simulink model "fdctools"  (Simulink 2.09)
settings: Solver=ode45  StartTime=0.0  StopTime=999999  MaxStep=10  RelTol=1e-3  AbsTol=1e-3
settings Model: SaveTime=off  SaveOutput=off  ConsistencyChecking=off  RTWTemplateMakefile=grt_vc.tmf

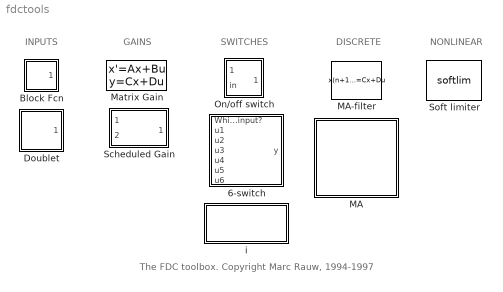
== system fdctools ==
  note: The FDC toolbox. Copyright Marc Rauw, 1994-1997
  note: GAINS
  note: SWITCHES
  note: DISCRETE
  note: NONLINEAR
  note: INPUTS
  6-switch : Subsystem
      mask Display: disp('6 switch:\ny=u(u[1]+1)')
  Block Fcn : Subsystem  mask(Block Fcn){@1=-1, @2=2, @3=1, @4=4}
      mask prompts: @1 "Initial value (=final value):"; @2 "Amplitude of block (+ = step up, - = step down):"; @3 "Start time of block:"; @4 "Stop time of block:"
      mask help: Block Function
      mask init:
      | yinit=@1; yblock=@2; tstart=@3; tstop=@4;
      mask Help: This block implements a block signal.\nDefine the initial (=final) value, the\namplitude of the block (positive\n= upwards, negative=downwards),\nthe start time, and the stop time (must\nbe smaller than the start time).
      mask Display: plot(0,0,100,100,[100,60,60,20,20,0],[50,50,89,89,50,50])
  Doublet : Subsystem  mask(Doublet){@1=1, @2=1, @3=1, @4=1, @5=-1, @6=0}
      mask prompts: @1 "Start time [sec]:"; @2 "Length of time interval 1 [sec]:"; @3 "Length of time interval 2 [sec]:"; @4 "y1:"; @5 "y2:"; @6 "y start (= y final):"
      mask help: Doublet signal.
      mask init:
      | ts1=@1; dt1=@2; dt2=@3; y1=@4; y2=@5; cnst=@6;
      mask Help: This block implements a \ndoublet signal according to: \ny = y1 if \n   tstart <= t < tstart+dt1 \ny = y2 if \n   tstart+dt1 <= t < tstart+dt1+dt2 \ny = y start = y final if \n   t < tstart or t > tstart+dt1+dt2.
      mask Display: plot([0 1 1 2.5 2.5 4 4 5],[0 0 1 1 -1.5 -1.5 0 0])
  MA : Subsystem
      mask Display: disp('MA filter\nwith better\nicon\n\n(double click)')
  MA-filter : DiscreteStateSpace  A=Ama  B=Bma  C=Cma  D=Dma  X0=xinit  SampleTime=Ts  mask(MA-filter){@1=5, @2=0.1, @3=0}
      mask prompts: @1 "Number of samples for averaging:"; @2 "Sample time:"; @3 "Initial value of input signal:"
      mask help: Digital Moving Average filter
      mask init:
      | ns=@1; Ama=[zeros(1,ns);[eye(ns-1) zeros(ns-1,1)]]; Bma=[1; zeros(ns-1,1)]; Cma=1/ns*ones(1,ns); Dma=0; Ts=@2; uinit=@3; xinit=uinit*ones(ns,1);
      mask Help: Digital Moving Average filter. \ny(k) = 1/n * (u(k) + u(k-1) + ... + u(k-ns)) \nwhere ns is the number of samples \nfor averaging (to be specified by \nthe user).
      mask Display: disp('MA')
  Matrix Gain : StateSpace  A=A  B=B  C=C  D=D  X0=0  mask(Matrix Gain){@1=eye(3)}
      mask prompts: @1 "Gain matrix:"
      mask help: Matrix Gain
      mask init:
      | A=[]; B=[]; C=[]; D=@1;
      mask Help: This block implements an matrix gain.\nThe matrix dimensions must be in accordance\nwith the dimension of the inputvector.
      mask Display: disp('y = M*u')
  On/off switch : Subsystem
      mask Type: On/off switch
      mask Description:
      | If input(1) = 1
      |      output = input(2)
      |  else if input(1) = 0
      |      output = 0
      mask Help: On/off switch.
      mask Display: plot(0,0,100,100,[31,31,32,34,34,32,31,31,0],[50,48,47,48,51,53,51,50,50],[100,75,51],[50,50,97]);disp('?')
  Scheduled Gain : Subsystem
      mask Display: plot(0,0,100,100,[0,100,0],[0,50,100]);disp('K(u1)      ')
  Soft limiter : S-Function  FunctionName=softlim  Parameters=max_u, lin_u  mask(Soft limiter){@1=10, @2=10}
      mask prompts: @1 "Limiter range= max. output value= --(min. output value):"; @2 "% of linear range where y=u (linear throughput):"
      mask help: Soft limiter with partly linear throughput
      mask init:
      | max_u=max(@1,1e-16); lin_u=min(0.9999,(max(@2,0)/100))*max_u; uplot=[-5*max_u:0.25*max_u:5*max_u]; for i = 1:length(uplot); yplot(i)=softlim([],[],uplot(i),3,max_u,lin_u); end;
      mask Help: See source-code of SOFTLIM.M or type HELP SOFTLIM at the command-line.
      mask Display: plot(uplot, yplot, max_u*[-5,-1,1,5], max_u*[-1,-1,1,1], 0, -1.3*max_u, 0, 1.2*max_u, max_u*[-5,5], [0,0]);
  i : Subsystem
      settings: OpenFcn=fdchelp('nswitch')
      mask Display: disp('More info\nfor n-switch')

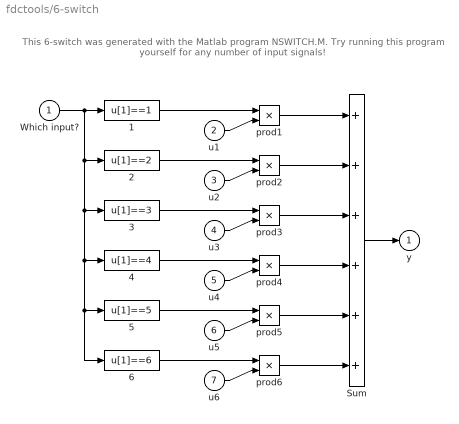
== system fdctools/6-switch ==
  note: This 6-switch was generated with the Matlab program NSWITCH.M.
      | Try running this program yourself for any number of input signals!
  Which input? : Inport  Port=1  PortWidth=-1  SampleTime=-1
  u1 : Inport  Port=2  PortWidth=-1  SampleTime=-1
  u2 : Inport  Port=3  PortWidth=-1  SampleTime=-1
  u3 : Inport  Port=4  PortWidth=-1  SampleTime=-1
  u4 : Inport  Port=5  PortWidth=-1  SampleTime=-1
  u5 : Inport  Port=6  PortWidth=-1  SampleTime=-1
  u6 : Inport  Port=7  PortWidth=-1  SampleTime=-1
  1 : Fcn  Expr=u[1]==1
  2 : Fcn  Expr=u[1]==2
  3 : Fcn  Expr=u[1]==3
  4 : Fcn  Expr=u[1]==4
  5 : Fcn  Expr=u[1]==5
  6 : Fcn  Expr=u[1]==6
  Sum : Sum  Inputs=++++++
  prod{1..6} (6 alike) : Product  Inputs=2
  y : Outport  Port=1  InitialOutput=0
  wires:
  Which input?/1 -> 1/1, 2/1, 3/1, 4/1, 5/1, 6/1
  u1/1 -> prod1/2
  prod1/1 -> Sum/1
  1/1 -> prod1/1
  u2/1 -> prod2/2
  prod2/1 -> Sum/2
  2/1 -> prod2/1
  u3/1 -> prod3/2
  prod3/1 -> Sum/3
  3/1 -> prod3/1
  u4/1 -> prod4/2
  prod4/1 -> Sum/4
  4/1 -> prod4/1
  u5/1 -> prod5/2
  prod5/1 -> Sum/5
  5/1 -> prod5/1
  u6/1 -> prod6/2
  prod6/1 -> Sum/6
  6/1 -> prod6/1
  Sum/1 -> y/1

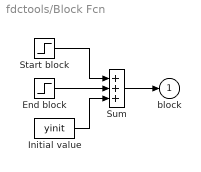
== system fdctools/Block Fcn ==
  End block : Step  Time=tstop  Before=0  After=-yblock
  Initial value : Constant  Value=yinit
  Start block : Step  Time=tstart  Before=0  After=yblock
  Sum : Sum  Inputs=+++
  block : Outport  Port=1  InitialOutput=0
  wires:
  Sum/1 -> block/1
  Initial value/1 -> Sum/3
  Start block/1 -> Sum/1
  End block/1 -> Sum/2

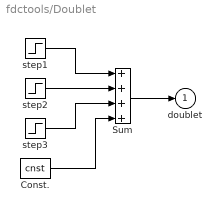
== system fdctools/Doublet ==
  Const. : Constant  Value=cnst
  Sum : Sum  Inputs=++++
  step1 : Step  Time=ts1  Before=0  After=y1-cnst
  step2 : Step  Time=ts1+dt1  Before=0  After=-y1+y2
  step3 : Step  Time=ts1+dt1+dt2  Before=0  After=-y2+cnst
  doublet : Outport  Port=1  InitialOutput=0
  wires:
  Const./1 -> Sum/4
  Sum/1 -> doublet/1
  step1/1 -> Sum/1
  step2/1 -> Sum/2
  step3/1 -> Sum/3

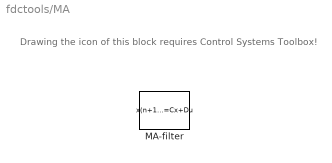
== system fdctools/MA ==
  note: Drawing the icon of this
      | block requires Control
      | Systems Toolbox!
  MA-filter : DiscreteStateSpace  A=Ama  B=Bma  C=Cma  D=Dma  X0=xinit  SampleTime=Ts  mask(MA-filter){ns=5, Ts=0.1, uinit=0}
      mask prompts: ns "Number of samples for averaging:"; Ts "Sample time:"; uinit "Initial value of input signal:"
      mask help: Digital Moving Average filter
      mask init:
      | Ama=[zeros(1,ns);[eye(ns-1) zeros(ns-1,1)]]; Bma=[1; zeros(ns-1,1)]; Cma=1/ns*ones(1,ns); Dma=0; xinit=uinit*ones(ns,1);  y=dstep(Ama,Bma,Cma,Dma,1,ns*1.5); yy=[]; for i = 1:length(y)-1; yy=[yy y(i) y(i+1)]; tt=[tt i i]; end; ly=length(y);
      mask Help: Digital Moving Average filter. \ny(k) = 1/n * (u(k) + u(k-1) + ... + u(k-ns)) \nwhere ns is the number of samples \nfor averaging (to be specified by \nthe user).
      mask Display: plot(tt,yy,[-0.3*ly 0 0 ly],[0 0 1 1],[0 1],[0 0],-0.3*ly-1,-0.25,ly+1,1.25)

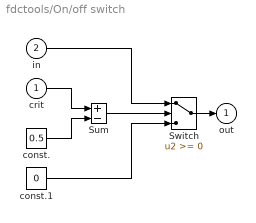
== system fdctools/On/off switch ==
  crit : Inport  Port=1  PortWidth=-1  SampleTime=-1
  in : Inport  Port=2  PortWidth=-1  SampleTime=-1
  Sum : Sum  Inputs=+-
  Switch : Switch  Threshold=0
  const. : Constant  Value=0.5
  const.1 : Constant  Value=0
  out : Outport  Port=1  InitialOutput=0
  wires:
  crit/1 -> Sum/1
  const.1/1 -> Switch/3
  Sum/1 -> Switch/2
  Switch/1 -> out/1
  in/1 -> Switch/1
  const./1 -> Sum/2

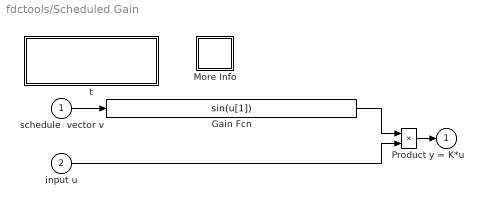
== system fdctools/Scheduled Gain ==
  schedule  vector v : Inport  Port=1  PortWidth=-1  SampleTime=-1
  input u : Inport  Port=2  PortWidth=-1  SampleTime=-1
  Gain Fcn : Fcn  Expr=sin(u[1])
  More Info : Subsystem
      mask Display: disp('???')
  Product : Product  Inputs=2
  t : Subsystem
      mask Display: disp('Scheduled Gain\nMarc Rauw\nAugust 1996')
  y = K*u : Outport  Port=1  InitialOutput=0
  wires:
  schedule  vector v/1 -> Gain Fcn/1
  Product/1 -> y = K*u/1
  input u/1 -> Product/2
  Gain Fcn/1 -> Product/1

== system fdctools/i ==
  note: Run NSWITCH.M to generate an n-switch with a
      | different number of inputs. Type HELP NSWITCH
      | at the Matlab command line for more info.

== system fdctools/Scheduled Gain/More Info ==
  note: The first input is the schedule signal. Change the
      | Gain Function to the required gain scheduling function.
  note: Scheduled Gain.
      |
      | Input 2 is multiplied with a gain which is a function
      | of input(-vector) 1. The schedule function should be
      | specified in the block 'Gain Fcn'.

== system fdctools/Scheduled Gain/t ==
